simulink model "test_modelu"  (R2016a)
settings: Solver=VariableStepAuto  StartTime=0.0  StopTime=10.0  RelTol=1e-3
values from neighbouring files (symbols this model uses):
  A_dw = 110.74    [zmienne.m]
  A_fm = 59900/3    (= 19966.6666667)    [zmienne.m]
  A_fs = 60.67    [zmienne.m]
  A_p = (PI * (D_i^2) * N) / (4 * 144)    (= 11.0984259136)    [zmienne.m]
  alfa_c = -2.0 * 10^-4    (= -0.0002)    [zmienne.m]
  alfa_f = -1.1 * 10^-5    (= -1.1e-05)    [zmienne.m]
  B_1 = 0.000209    [zmienne.m]
  B_2 = 0.001414    [zmienne.m]
  B_3 = 0.001309    [zmienne.m]
  B_4 = 0.002727    [zmienne.m]
  B_5 = 0.000925    [zmienne.m]
  B_6 = 0.000314    [zmienne.m]
  B_t = 0.00689    [zmienne.m]
  C_1 = 1 / sqrt(C_d)    [zmienne.m]
  C_m = 0.11    [zmienne.m]
  C_p1 = 1.39    [zmienne.m]
  C_p2 = 1.165    [zmienne.m]
  C_pf = 0.059    [zmienne.m]
  C_pmo = 1.39    [zmienne.m]
  CP_fw = 1.218    [zmienne.m]
  DENS_d = 50.32    [zmienne.m]
  DENS_dw = 47.66    [zmienne.m]
  DENS_s = 52.32    [zmienne.m]
  DENS_w = 45.710    (= 45.71)    [zmienne.m]
  F_r = 0.974    [zmienne.m]
  G_1 = 65.2    [zmienne.m]
  G_2 = 1.0    (= 1)    [zmienne.m]
  G_v = 32.2    [zmienne.m]
  H_fm = 200/3600    (= 0.0555555555556)    [zmienne.m]
  K1 = 3.5 * 10^-6    (= 3.5e-06)    [zmienne.m]
  K2 = -7.135 * 10^-4    (= -0.0007135)    [zmienne.m]
  K3 = 0.17    [zmienne.m]
  K4 = -0.2    [zmienne.m]
  K5 = 0.14    [zmienne.m]
  K7 = 2.37 * 10^-3    (= 0.00237)    [zmienne.m]
  K9 = -0.035    [zmienne.m]
  L = 35.54    [zmienne.m]
  L_d = 35.54    [zmienne.m]
  L_dw0 = 9.63    [zmienne.m]
  L_r = 9.63    [zmienne.m]
  lambda_1 = 0.0125    [zmienne.m]
  lambda_2 = 0.0308    [zmienne.m]
  lambda_3 = 0.114    [zmienne.m]
  lambda_4 = 0.307    [zmienne.m]
  lambda_5 = 1.19    [zmienne.m]
  lambda_6 = 3.19    [zmienne.m]
  m0 = 0    [zmienne.m]
  M_d = DENS_d * A_d *L_d    (= 57227.9296)    [zmienne.m]
  M_f = M_ft * 3    (= 668217)    [zmienne.m]
  M_m1 = (M_m * L_s10) / L    (= 5577.64460636)    [zmienne.m]
  M_m2 = M_m * (L_s20 / L)    (= 51851.8797758)    [zmienne.m]
  M_m3 = M_m2    (= 51851.8797758)    [zmienne.m]
  M_m4 = M_m1    (= 5577.64460636)    [zmienne.m]
  M_mo = V_mo * DENS_mo / 3    (= 8227.8)    [zmienne.m]
  M_p1 = (M_p * L_s10) / L    (= 1751.07864275)    [zmienne.m]
  M_p2 = (M_p * L_s20) / L    (= 16278.6849414)    [zmienne.m]
  NGT = 17.9 * 10^-6    (= 1.79e-05)    [zmienne.m]
  P_0 = (P_cor10 * 3.41) / (3600 * 3)    (= 1084885.18519)    [zmienne.m]
  P_r2 = S_pm2 / L_s20    (= 687.386379167)    [zmienne.m]
  POWER_i = 691244.4199    [zmienne.m]
  r0 = 0    [zmienne.m]
  S_ms1 = S_m * (L_s10 / L)    (= 2678.800154)    [zmienne.m]
  S_ms2 = S_m * (L_s20 / L)    (= 24903.1326539)    [zmienne.m]
  S_ms3 = S_ms2    (= 24903.1326539)    [zmienne.m]
  S_ms4 = S_ms1    (= 2678.800154)    [zmienne.m]
  S_pm1 = (S_ms1 * D_i) / D_o    (= 2372.65156497)    [zmienne.m]
  S_pm2 = (S_ms2 * D_i) / D_o    (= 22057.0603506)    [zmienne.m]
  S_pm3 = S_pm1    (= 2372.65156497)    [zmienne.m]
  S_pm4 = S_pm2    (= 22057.0603506)    [zmienne.m]
  T_f10 = 1488.75    [zmienne.m]
  T_f20 = 1506.38    [zmienne.m]
  T_f30 = 1523.96    [zmienne.m]
  T_mo10 = 548.303    [zmienne.m]
  T_mo20 = 557.106    [zmienne.m]
  T_mo30 = 565.909    [zmienne.m]
  T_mo40 = 574.711    [zmienne.m]
  T_mo50 = 583.514    [zmienne.m]
  T_mo60 = 592.5    [zmienne.m]
  tau = 5    [zmienne.m]
  tau_1 = 250    [zmienne.m]
  tau_2 = 120    [zmienne.m]
  tau_cl = M_cl / W_pt    (= 2.08881752232)    [zmienne.m]
  tau_hl = M_hl / W_pt    (= 1.04440876116)    [zmienne.m]
  tau_la1 = 10    [zmienne.m]
  tau_la2 = 5    [zmienne.m]
  tau_le = 80    [zmienne.m]
  tau_lp = M_lp / W_pt    (= 1.87053609124)    [zmienne.m]
  tau_mo = M_mo / (2 * W_pt)    (= 0.0939967885046)    [zmienne.m]
  tau_pi = M_pi / W_pi    (= 0.60183806901)    [zmienne.m]
  tau_rtd = 4    [zmienne.m]
  tau_set = 30    [zmienne.m]
  tau_up = M_up / W_pt    (= 1.43710645536)    [zmienne.m]
  U_ms1 = 1 / (((1 / h_os) + (D_o * log(D_o/D_m))) / (24 * K_th))    [zmienne.m]
  U_ms2 = 1 / (((1 / h_ob) + (D_o * log(D_o/D_m))) / (24 * K_th))    [zmienne.m]
  U_pm = 1 / (((1 / h_i) + (D_i * log(D_m/D_i))) / (24 * K_th))    [zmienne.m]
  V_dr = 4398.706    [zmienne.m]
  V_r = 468.981    [zmienne.m]
  w0 = 0    [zmienne.m]
  W_fi0 = 1036.39    [zmienne.m]
  W_nv = 0.63    [zmienne.m]
  W_pi = 10941.6    [zmienne.m]
  X1 = 402.94    [zmienne.m]
  X2 = 0.018    [zmienne.m]
  X3 = 1.13096    [zmienne.m]
  X4 = 370.751    [zmienne.m]
  X5 = 850.04    [zmienne.m]
  X6 = -0.181289    [zmienne.m]
  X8 = 1225.85    [zmienne.m]
  Z_tv = 3.18    [zmienne.m]
undefined symbols (not defined in the file or in its folder): magnitude
(part 1 of 2)
settings Model: Creator=Użytkownik  LastModifiedBy=Użytkownik
settings GRTTargetCC: GeneratePreprocessorConditionals=Use local settings

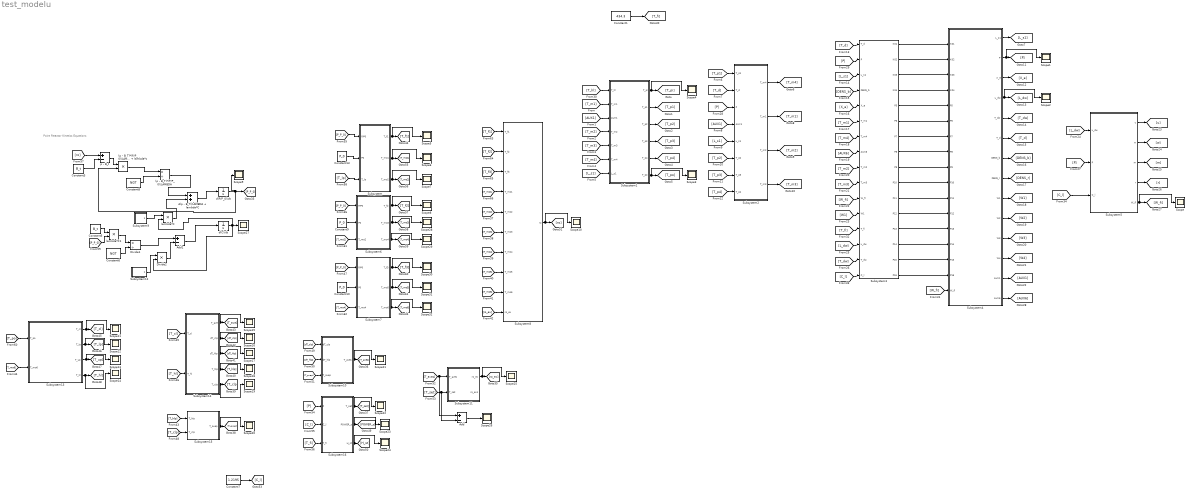
== system test_modelu ==
  note: Point Reactor Kinetics Equations
  (p - B_T)*(P/P_0)/LAMBDA : Product  Inputs=*/
  (p - B_T)*(P/P_0)/LAMBDA + lambda*c : Product  Inputs=**
  A(p - B_T)/LAMBDA + lambda*C : Sum
  Add : Sum  Inputs=+-
  Add1 : Sum  Inputs=+-
  Constant1 : Constant  Value=434.3
  Constant10 : Constant  Value=P_0
  Constant13 : Constant  Value=P_0
  Constant3 : Constant  Value=B_t
  Constant5 : Constant  Value=B_t
  Constant6 : Constant  Value=NGT
  Constant7 : Constant  Value=1.2195
  Constant8 : Constant  Value=NGT
  Constant9 : Constant  Value=P_0
  Divide1 : Product  Inputs=*/
  Divide2 : Product  Inputs=**
  Scope{,1..32} (33 alike) : Scope
  Subsystem : Subsystem
  Subsystem1 : Subsystem
  Subsystem10 : Subsystem
  Subsystem11 : Subsystem
  Subsystem12 : Subsystem
  Subsystem13 : Subsystem
  Subsystem14 : Subsystem
  Subsystem15 : Subsystem
  Subsystem16 : Subsystem
  Subsystem2 : Subsystem
  Subsystem3 : Subsystem
  Subsystem4 : Subsystem
  Subsystem5 : Subsystem
  Subsystem6 : Subsystem
  Subsystem7 : Subsystem
  Subsystem8 : Subsystem
  Subsystem9 : Subsystem
  d(C)/dt : Integrator  InitialCondition=4625.71
  d(P/P_0)/dt : Integrator  InitialCondition=1
  lambda*C : Product  Inputs=**
  lambda*C1 : Product  Inputs=**
  p - B_t : Sum  Inputs=+-
  wires:
  Subsystem1/1(T_pi) -> Scope4/1, [T_pi]
  Subsystem1/2(T_p1) -> [T_p1]
  Subsystem1/3(T_p2) -> [T_p2]
  Subsystem1/4(T_p3) -> [T_p3]
  Subsystem1/5(T_p4) -> [T_p4]
  Subsystem1/6(T_po) -> Scope3/1, [T_po]
  Subsystem2/1(T_m4) -> [T_m4]
  Subsystem2/2(T_m1) -> [T_m1]
  Subsystem2/3(T_m2) -> [T_m2]
  Subsystem2/4(T_m3) -> [T_m3]
  Subsystem4/1(L_s1) -> [L_s1]
  Subsystem4/2(P) -> Scope1/1, [P]
  Subsystem4/3(X_e) -> [X_e]
  Subsystem4/4(L_dw) -> Scope2/1, [L_dw]
  Subsystem4/5(T_dw) -> [T_dw]
  Subsystem4/6(T_d) -> [T_d]
  Subsystem4/7(DENS_b) -> [DENS_b]
  Subsystem4/8(DENS_r) -> [DENS_r]
  Subsystem4/9(W1) -> [W1]
  Subsystem4/10(W2) -> [W2]
  Subsystem4/11(W3) -> [W3]
  Subsystem4/12(W4) -> [W4]
  Subsystem4/13(AUX1) -> [AUX1]
  [T_m1] -> Subsystem1/2(T_m1)
  [AUX1] -> Subsystem1/3(AUX1)
  [T_m2] -> Subsystem1/4(T_m2)
  [T_m3] -> Subsystem1/5(T_m3)
  [T_m4] -> Subsystem1/6(T_m4)
  [L_s1] -> Subsystem1/7(L_s1)
  Subsystem5/1(u) -> [u]
  Subsystem5/2(w) -> [w]
  Subsystem5/3(m) -> [m]
  Subsystem5/4(r) -> [r]
  Subsystem5/5(W_fi) -> Scope/1, [W_fi]
  [T_p1] -> Subsystem2/1(T_p1)
  [T_d] -> Subsystem2/2(T_d)
  [AUX1] -> Subsystem2/4(AUX1)
  [L_s1] -> Subsystem2/5(L_s1)
  [T_p2] -> Subsystem2/6(T_p2)
  [T_p3] -> Subsystem2/7(T_p3)
  [T_p4] -> Subsystem2/8(T_p4)
  [T_d] -> Subsystem3/1(T_d)
  [L_s1] -> Subsystem3/3(L_s1)
  [DENS_b] -> Subsystem3/4(DENS_b)
  [X_e] -> Subsystem3/5(X_e)
  [T_m1] -> Subsystem3/6(T_m1)
  [T_m4] -> Subsystem3/7(T_m4)
  [T_m2] -> Subsystem3/9(T_m2)
  [T_m3] -> Subsystem3/10(T_m3)
  [W_fi] -> Subsystem3/11(W_fi)
  [AUX6] -> Subsystem3/8(AUX6)
  Subsystem4/14(AUX6) -> [AUX6]
  [W1] -> Subsystem3/12(W1)
  [L_dw] -> Subsystem3/14(L_dw)
  [T_dw] -> Subsystem3/15(T_dw)
  [L_dw] -> Subsystem5/1(L_dw)
  [P] -> Subsystem5/2(P)
  [P] -> Subsystem2/3(P)
  [P] -> Subsystem3/2(P)
  [T_hl] -> Subsystem1/1(T_hl)
  [W_fi] -> Subsystem4/17(W_fi)
  [T_fi] -> Subsystem3/13(T_fi)
  [C_l] -> Subsystem3/16(C_l)
  [C_l] -> Subsystem5/3(C_l)
  Constant1/1 -> [T_fi]
  Subsystem3/1(K01) -> Subsystem4/1(K01)
  Subsystem3/2(K02) -> Subsystem4/2(K02)
  Subsystem3/3(K03) -> Subsystem4/3(K03)
  Subsystem3/4("K04 ") -> Subsystem4/4(K04)
  Subsystem3/5(P5) -> Subsystem4/5(P5)
  Subsystem3/6(P6) -> Subsystem4/6(P6)
  Subsystem3/7(P7) -> Subsystem4/7(P7)
  Subsystem3/8(P8) -> Subsystem4/8(P8)
  Subsystem3/9(P9) -> Subsystem4/9(P9)
  Subsystem3/10(P10) -> Subsystem4/10(P10)
  Subsystem3/11(P11) -> Subsystem4/11(P11)
  Subsystem3/12(P12) -> Subsystem4/12(P12)
  Subsystem3/13(P13) -> Subsystem4/13(P13)
  Subsystem3/14(P14) -> Subsystem4/14(P14)
  Subsystem3/15(P15) -> Subsystem4/15(P15)
  Subsystem3/16(P16) -> Subsystem4/16(P16)
  Constant3/1 -> p - B_t/2
  Constant8/1 -> (p - B_T)*(P/P_0)/LAMBDA/2
  Subsystem9/1(lambda) -> lambda*C/1
  d(C)/dt/1 -> Scope27/1, Divide2/2, lambda*C/2
  lambda*C/1 -> A(p - B_T)/LAMBDA + lambda*C/2
  A(p - B_T)/LAMBDA + lambda*C/1 -> d(P/P_0)/dt/1
  Constant6/1 -> Divide1/2
  Divide1/1 -> Add1/1
  Subsystem12/1(lambda) -> Divide2/1
  Divide2/1 -> Add1/2
  Add1/1 -> d(C)/dt/1
  d(P/P_0)/dt/1 -> (p - B_T)*(P/P_0)/LAMBDA + lambda*c/2, [P_P_0], Scope9/1
  Constant13/1 -> Subsystem/2(P0)
  Constant9/1 -> Subsystem6/2(P0)
  Constant10/1 -> Subsystem7/2(P0)
  [T_po] -> Subsystem13/1(T_po)
  [P_P_0] -> Subsystem/1("P/P0 ")
  [P_P_0] -> Subsystem6/1("P/P0 ")
  [P_P_0] -> Subsystem7/1("P/P0 ")
  Subsystem/1(T_f1) -> Scope5/1, [T_f1]
  Subsystem/2(T_mo1) -> Scope6/1, [T_mo1]
  Subsystem/3(T_mo2) -> Scope7/1, [T_mo2]
  Subsystem6/1(T_f2) -> Scope8/1, [T_f2]
  Subsystem6/2(T_mo3) -> Scope28/1, [T_mo3]
  Subsystem6/3(T_mo4) -> Scope29/1, [T_mo4]
  Subsystem7/1(T_f3) -> Scope30/1, [T_f3]
  Subsystem7/2(T_mo5) -> Scope31/1, [T_mo5]
  Subsystem7/3(T_mo6) -> Scope32/1, [T_mo6]
  [T_lp] -> Subsystem/3(T_lp)
  [T_mo2] -> Subsystem6/3(T_mo2)
  [T_mo4] -> Subsystem7/3(T_mo4)
  [T_f1] -> Subsystem8/1(T_f1)
  [T_f2] -> Subsystem8/2(T_f2)
  [T_f3] -> Subsystem8/3(T_f3)
  [T_mo1] -> Subsystem8/4(T_mo1)
  [T_mo2] -> Subsystem8/5(T_mo2)
  [T_mo3] -> Subsystem8/6(T_mo3)
  [T_mo4] -> Subsystem8/7(T_mo4)
  [T_mo5] -> Subsystem8/8(T_mo5)
  [T_mo6] -> Subsystem8/9(T_mo6)
  [ro_ex] -> Subsystem8/10(ro_ex)
  [T_cl] -> Subsystem14/1(T_cl)
  [T_hl] -> Subsystem14/2(T_hl)
  [T_hlp] -> Subsystem15/1(T_hlp)
  [T_clp] -> Subsystem15/2(T_clp)
  [dT_clp] -> Subsystem10/1(dT_clp)
  [dT_hlp] -> Subsystem10/2(dT_hlp)
  [T_avep] -> Subsystem10/3(T_avep)
  [T_aves] -> Add/1, Subsystem11/1(T_aves)
  [T_set] -> Add/2, Subsystem11/2(T_set)
  Subsystem10/1(T_aves) -> Scope21/1, [T_aves]
  Subsystem16/1(T_set) -> Scope22/1, [T_set]
  Subsystem15/1(T_avep) -> Scope20/1, [T_avep]
  Subsystem14/5(T_clp) -> Scope19/1, [T_clp]
  Subsystem14/4(T_hlp) -> Scope18/1, [T_hlp]
  Subsystem14/3(dT_hlp) -> Scope17/1, [dT_hlp]
  Subsystem14/2(dT_clp) -> Scope16/1, [dT_clp]
  Subsystem14/1(T_ave) -> Scope15/1, [T_ave]
  Subsystem13/3(T_up) -> Scope13/1, [T_up]
  Subsystem13/2(T_lp) -> Scope12/1, [T_lp]
  Subsystem13/1(T_cl) -> Scope11/1, [T_cl]
  Subsystem16/2(POWER_s) -> [POWER_s], Scope23/1
  [P] -> Subsystem16/1(P)
  [C_l] -> Subsystem16/2(C_l)
  [T_fi] -> Subsystem16/3(T_fi)
  [T_mo6] -> Subsystem13/2(T_mo6)
  Subsystem8/1(ro) -> Scope10/1, [ro]
  Constant7/1 -> [C_l]
  Constant5/1 -> lambda*C1/1
  [P_P_0] -> lambda*C1/2
  lambda*C1/1 -> Divide1/1
  Subsystem11/1(ro_ex) -> Scope25/1, [ro_ex]
  Subsystem16/3(H_st) -> Scope24/1, [H_st]
  Add/1 -> Scope26/1
  Subsystem13/4(T_hl) -> Scope14/1, [T_hl]
  p - B_t/1 -> (p - B_T)*(P/P_0)/LAMBDA + lambda*c/1
  (p - B_T)*(P/P_0)/LAMBDA + lambda*c/1 -> (p - B_T)*(P/P_0)/LAMBDA/1
  (p - B_T)*(P/P_0)/LAMBDA/1 -> A(p - B_T)/LAMBDA + lambda*C/1
  [ro] -> p - B_t/1

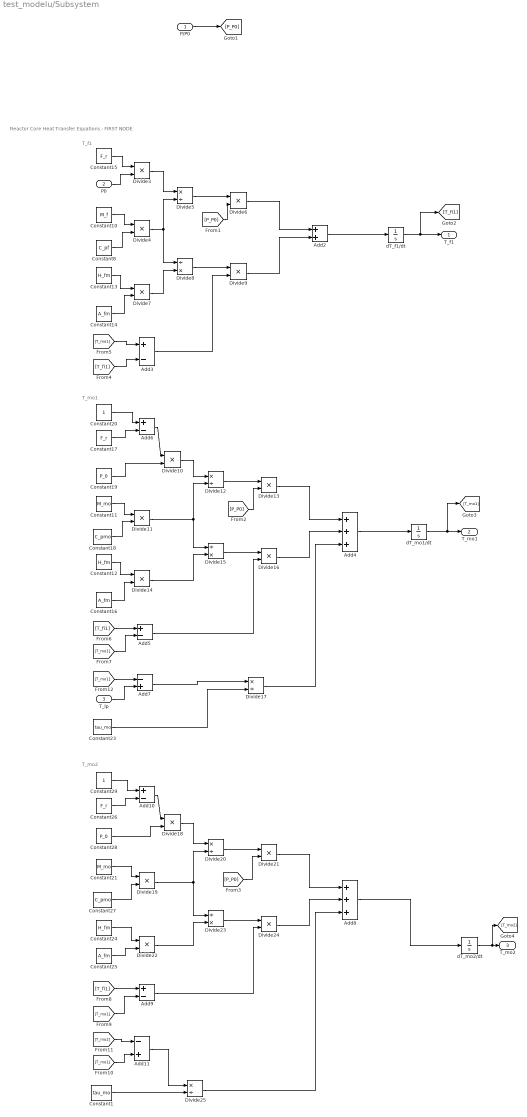
== system test_modelu/Subsystem ==
  note: T_mo2
  note: T_mo1
  note: T_f1
  note: Reactor Core Heat Transfer Equations : FIRST NODE
  "P/P0 " : Inport
  P0 : Inport  Port=2
  T_lp : Inport  Port=3
  Add{3,5..6,9..10} (5 alike) : Sum  Inputs=+-
  Add11 : Sum  Inputs=-+
  Add2 : Sum
  Add4 : Sum  Inputs=+++
  Add7 : Sum  Inputs=-+
  Add8 : Sum  Inputs=+++
  Constant1 : Constant  Value=tau_mo
  Constant10 : Constant  Value=M_f
  Constant11 : Constant  Value=M_mo
  Constant12 : Constant  Value=H_fm
  Constant13 : Constant  Value=H_fm
  Constant14 : Constant  Value=A_fm
  Constant15 : Constant  Value=F_r
  Constant16 : Constant  Value=A_fm
  Constant17 : Constant  Value=F_r
  Constant18 : Constant  Value=C_pmo
  Constant19 : Constant  Value=P_0
  Constant20 : Constant
  Constant21 : Constant  Value=M_mo
  Constant23 : Constant  Value=tau_mo
  Constant24 : Constant  Value=H_fm
  Constant25 : Constant  Value=A_fm
  Constant26 : Constant  Value=F_r
  Constant27 : Constant  Value=C_pmo
  Constant28 : Constant  Value=P_0
  Constant29 : Constant
  Constant8 : Constant  Value=C_pf
  Divide{3..4,6..7,9..11,13..14,16,18..19,21..22,24} (15 alike) : Product  Inputs=**
  Divide{5,12,17,20,25} (5 alike) : Product  Inputs=*/
  Divide15 : Product  Inputs=/*
  Divide23 : Product  Inputs=/*
  Divide8 : Product  Inputs=/*
  dT_f1/dt : Integrator  InitialCondition=1488.75
  dT_mo1/dt : Integrator  InitialCondition=548.303
  dT_mo2/dt : Integrator  InitialCondition=557.106
  T_f1 : Outport
  T_mo1 : Outport  Port=2
  T_mo2 : Outport  Port=3
  wires:
  Constant15/1 -> Divide3/1
  Constant10/1 -> Divide4/1
  Constant8/1 -> Divide4/2
  Divide3/1 -> Divide5/1
  Divide4/1 -> Divide5/2, Divide8/1
  Divide5/1 -> Divide6/1
  Divide6/1 -> Add2/1
  Constant13/1 -> Divide7/1
  Constant14/1 -> Divide7/2
  Divide7/1 -> Divide8/2
  Divide8/1 -> Divide9/1
  dT_mo1/dt/1 -> [T_mo1], T_mo1/1
  dT_f1/dt/1 -> [T_fi1], T_f1/1
  Add3/1 -> Divide9/2
  Divide9/1 -> Add2/2
  Add2/1 -> dT_f1/dt/1
  Constant19/1 -> Divide10/2
  Constant11/1 -> Divide11/1
  Constant18/1 -> Divide11/2
  Divide10/1 -> Divide12/1
  Divide11/1 -> Divide15/1, Divide12/2
  Divide12/1 -> Divide13/1
  Divide13/1 -> Add4/1
  Constant12/1 -> Divide14/1
  Constant16/1 -> Divide14/2
  Divide14/1 -> Divide15/2
  Divide15/1 -> Divide16/1
  Add5/1 -> Divide16/2
  Divide16/1 -> Add4/2
  Constant20/1 -> Add6/1
  Constant17/1 -> Add6/2
  Add6/1 -> Divide10/1
  T_lp/1 -> Add7/2
  Add7/1 -> Divide17/1
  Constant23/1 -> Divide17/2
  Divide17/1 -> Add4/3
  Add4/1 -> dT_mo1/dt/1
  dT_mo2/dt/1 -> [T_mo2], T_mo2/1
  Constant28/1 -> Divide18/2
  Constant21/1 -> Divide19/1
  Constant27/1 -> Divide19/2
  Divide18/1 -> Divide20/1
  Divide19/1 -> Divide20/2, Divide23/1
  Divide20/1 -> Divide21/1
  Divide21/1 -> Add8/1
  Constant24/1 -> Divide22/1
  Constant25/1 -> Divide22/2
  Divide22/1 -> Divide23/2
  Divide23/1 -> Divide24/1
  Add9/1 -> Divide24/2
  Divide24/1 -> Add8/2
  Constant29/1 -> Add10/1
  Constant26/1 -> Add10/2
  Add10/1 -> Divide18/1
  Add11/1 -> Divide25/1
  Divide25/1 -> Add8/3
  Add8/1 -> dT_mo2/dt/1
  "P/P0 "/1 -> [P_P0]
  P0/1 -> Divide3/2
  [P_P0] -> Divide6/2
  [P_P0] -> Divide21/2
  [P_P0] -> Divide13/2
  [T_mo1] -> Add3/1
  [T_fi1] -> Add3/2
  [T_fi1] -> Add5/1
  [T_mo1] -> Add5/2
  [T_fi1] -> Add9/1
  [T_mo1] -> Add9/2
  [T_mo2] -> Add11/1
  [T_mo1] -> Add11/2
  [T_mo1] -> Add7/1
  Constant1/1 -> Divide25/2

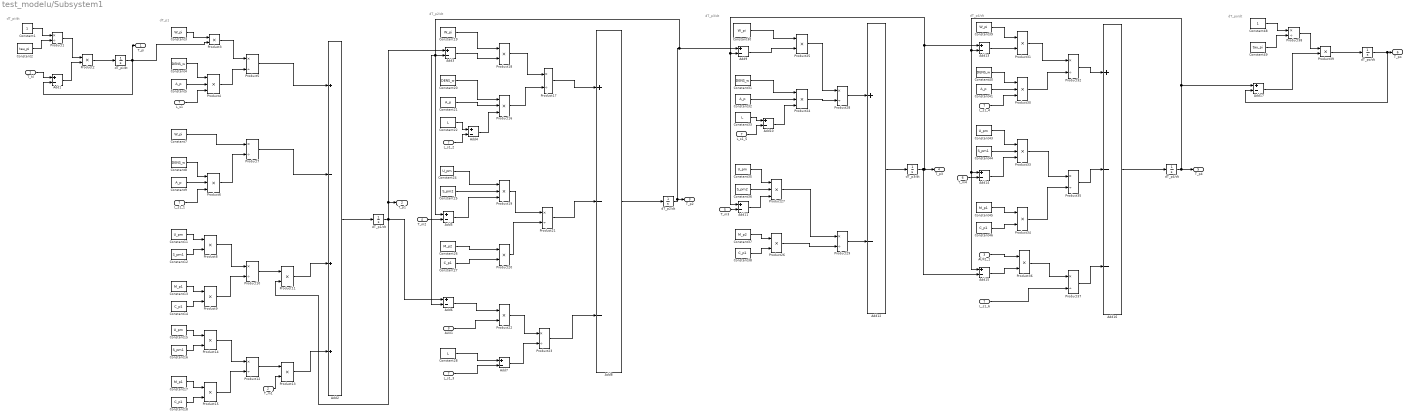
== system test_modelu/Subsystem1 ==
  note: dT_po/dt
  note: dT_p4/dt
  note: dT_p3/dt
  note: dT_p2/dt
  note: dT_p1
  note: dT_pi/dt
  T_hl : Inport
  T_m1 : Inport  Port=2
  AUX1 : Inport  Port=3
  T_m2 : Inport  Port=4
  T_m3 : Inport  Port=5
  T_m4 : Inport  Port=6
  L_s1 : Inport  Port=7
  AUX1_1 : InportShadow  Port=3
  Add{1,3..7,9..15,17} (14 alike) : Sum  Inputs=+-
  Add16 : Sum  Inputs=+--
  Add2 : Sum  Inputs=+-++
  Add8 : Sum  Inputs=+--
  Constant1 : Constant
  Constant{11,15,24,35,43} (5 alike) : Constant  Value=U_pm
  Constant12 : Constant  Value=S_pm1
  Constant13 : Constant  Value=M_p1
  Constant{14,18,27,38,46} (5 alike) : Constant  Value=C_p1
  Constant16 : Constant  Value=S_pm1
  Constant17 : Constant  Value=M_p1
  Constant{3,7,19,30,39} (5 alike) : Constant  Value=W_pi
  Constant2 : Constant  Value=tau_pi
  Constant{4,8,20,31,40} (5 alike) : Constant  Value=DENS_w
  Constant{5,9,21,32,41} (5 alike) : Constant  Value=A_p
  Constant22 : Constant  Value=L
  Constant25 : Constant  Value=S_pm2
  Constant26 : Constant  Value=M_p2
  Constant28 : Constant  Value=L
  Constant33 : Constant  Value=L
  Constant36 : Constant  Value=S_pm2
  Constant37 : Constant  Value=M_p2
  Constant44 : Constant  Value=S_pm1
  Constant45 : Constant  Value=M_p1
  Constant48 : Constant
  Constant49 : Constant  Value=tau_pi
  L_s1_{1..6} (6 alike) : InportShadow  Port=7
  Product{1,5,7,10,12,17,21,23,28..29,32,35,37..38} (14 alike) : Product  Inputs=*/
  Product{2..3,8..9,11,13..15,18,20,22,25..26,31,34,36,39} (17 alike) : Product
  Product{4,6,16,19,24,27,30,33} (8 alike) : Product  Inputs=3
  dT_p1/dt : Integrator  InitialCondition=587.36
  dT_p2/dt : Integrator  InitialCondition=557.4
  dT_p3/dt : Integrator  InitialCondition=542.5
  dT_p4/dt : Integrator  InitialCondition=539.5
  dT_pi/dt : Integrator  InitialCondition=592.5
  dT_po/dt : Integrator  InitialCondition=539.5
  T_pi : Outport
  T_p1 : Outport  Port=2
  T_p2 : Outport  Port=3
  T_p3 : Outport  Port=4
  T_p4 : Outport  Port=5
  T_po : Outport  Port=6
  wires:
  Constant1/1 -> Product1/1
  Constant2/1 -> Product1/2
  T_hl/1 -> Add1/1
  Product1/1 -> Product2/1
  Add1/1 -> Product2/2
  Product2/1 -> dT_pi/dt/1
  dT_pi/dt/1 -> T_pi/1, Product3/2, Add1/2
  Constant3/1 -> Product3/1
  Constant4/1 -> Product4/1
  Constant5/1 -> Product4/2
  L_s1/1 -> Product4/3
  Product3/1 -> Product5/1
  Product4/1 -> Product5/2
  Constant8/1 -> Product6/1
  Constant9/1 -> Product6/2
  L_s1_1/1 -> Product6/3
  Constant7/1 -> Product7/1
  Product6/1 -> Product7/2
  Constant11/1 -> Product8/1
  Constant12/1 -> Product8/2
  Constant13/1 -> Product9/1
  Constant14/1 -> Product9/2
  Product8/1 -> Product10/1
  Product9/1 -> Product10/2
  Product10/1 -> Product11/1
  Constant15/1 -> Product14/1
  Constant16/1 -> Product14/2
  Constant17/1 -> Product15/1
  Constant18/1 -> Product15/2
  Product14/1 -> Product12/1
  Product15/1 -> Product12/2
  Product12/1 -> Product13/1
  T_m1/1 -> Product13/2
  Product5/1 -> Add2/1
  Product7/1 -> Add2/2
  Product11/1 -> Add2/3
  Product13/1 -> Add2/4
  dT_p1/dt/1 -> Add6/1, Product11/2, T_p1/1, Add3/1
  Add2/1 -> dT_p1/dt/1
  Constant22/1 -> Add4/1
  L_s1_2/1 -> Add4/2
  Constant20/1 -> Product16/1
  Constant21/1 -> Product16/2
  Add4/1 -> Product16/3
  Constant19/1 -> Product18/1
  Add3/1 -> Product18/2
  Product18/1 -> Product17/1
  Product16/1 -> Product17/2
  Add5/1 -> Product19/3
  Constant25/1 -> Product19/2
  Constant24/1 -> Product19/1
  Constant26/1 -> Product20/1
  Constant27/1 -> Product20/2
  Product19/1 -> Product21/1
  Product20/1 -> Product21/2
  dT_p2/dt/1 -> T_p2/1, Add5/1, Add3/2, Add6/2, Add9/1
  Add6/1 -> Product22/1
  AUX1/1 -> Product22/2
  Constant28/1 -> Add7/1
  L_s1_3/1 -> Add7/2
  Product22/1 -> Product23/1
  Add7/1 -> Product23/2
  Add8/1 -> dT_p2/dt/1
  Product17/1 -> Add8/1
  Product21/1 -> Add8/2
  Product23/1 -> Add8/3
  Constant33/1 -> Add10/1
  L_s1_5/1 -> Add10/2
  Constant31/1 -> Product24/1
  Constant32/1 -> Product24/2
  Add10/1 -> Product24/3
  Constant30/1 -> Product25/1
  Add9/1 -> Product25/2
  dT_p3/dt/1 -> T_p3/1, Add11/1, Add9/2, Add13/1, Add15/2
  Constant37/1 -> Product26/1
  Constant38/1 -> Product26/2
  Constant35/1 -> Product27/1
  Constant36/1 -> Product27/2
  Add11/1 -> Product27/3
  T_m2/1 -> Add5/2
  T_m3/1 -> Add11/2
  Add12/1 -> dT_p3/dt/1
  Product28/1 -> Add12/1
  Product25/1 -> Product28/1
  Product24/1 -> Product28/2
  Product29/1 -> Add12/2
  Product27/1 -> Product29/1
  Product26/1 -> Product29/2
  dT_p4/dt/1 -> T_p4/1, Add17/1, Add15/1, Add14/1, Add13/2
  Constant41/1 -> Product30/2
  Constant40/1 -> Product30/1
  L_s1_4/1 -> Product30/3
  Constant39/1 -> Product31/1
  Add13/1 -> Product31/2
  Product31/1 -> Product32/1
  Product30/1 -> Product32/2
  T_m4/1 -> Add14/2
  Constant43/1 -> Product33/1
  Constant44/1 -> Product33/2
  Add14/1 -> Product33/3
  Constant45/1 -> Product34/1
  Constant46/1 -> Product34/2
  Product33/1 -> Product35/1
  Product34/1 -> Product35/2
  AUX1_1/1 -> Product36/1
  Add15/1 -> Product36/2
  Product36/1 -> Product37/1
  L_s1_6/1 -> Product37/2
  Add16/1 -> dT_p4/dt/1
  Product32/1 -> Add16/1
  Product35/1 -> Add16/2
  Product37/1 -> Add16/3
  Constant48/1 -> Product38/1
  Constant49/1 -> Product38/2
  dT_po/dt/1 -> Add17/2, T_po/1
  Product38/1 -> Product39/1
  Add17/1 -> Product39/2
  Product39/1 -> dT_po/dt/1

== system test_modelu/Subsystem10 ==
  dT_clp : Inport
  dT_hlp : Inport  Port=2
  T_avep : Inport  Port=3
  Add : Sum  Inputs=+--+
  Add1 : Sum
  Add2 : Sum
  Constant1 : Constant  Value=tau_la1
  Constant2 : Constant  Value=tau_la2
  Constant3 : Constant  Value=tau_le
  Constant4 : Constant  Value=2
  Constant5 : Constant  Value=tau_la1
  Constant6 : Constant  Value=tau_la2
  Divide : Product  Inputs=*/
  Divide1 : Product  Inputs=**
  Divide2 : Product  Inputs=*/
  Divide3 : Product  Inputs=**
  Divide4 : Product  Inputs=**
  dT_aves/dt : Integrator  InitialCondition=566
  d^2T_aves/dt : Integrator
  T_aves : Outport
  wires:
  T_avep/1 -> Add/1
  dT_aves/dt/1 -> [T_aves], T_aves/1
  Constant1/1 -> Add1/1
  Constant2/1 -> Add1/2
  Add1/1 -> Divide1/1
  d^2T_aves/dt/1 -> [AUX_co], dT_aves/dt/1
  Divide1/1 -> Add/3
  dT_clp/1 -> Add2/1
  dT_hlp/1 -> Add2/2
  Add2/1 -> Divide2/1
  Constant4/1 -> Divide2/2
  Constant3/1 -> Divide3/1
  Divide2/1 -> Divide3/2
  Divide3/1 -> Add/4
  Constant5/1 -> Divide4/1
  Constant6/1 -> Divide4/2
  Divide4/1 -> Divide/2
  Add/1 -> Divide/1
  Divide/1 -> d^2T_aves/dt/1
  [AUX_co] -> Divide1/2
  [T_aves] -> Add/2

== system test_modelu/Subsystem11 ==
  T_aves : Inport
  T_set : Inport  Port=2
  Integrator : Integrator
  MATLAB Function : MATLAB Function  TreatAsAtomicUnit=on
  MATLAB Function1 : MATLAB Function  TreatAsAtomicUnit=on
  Scope : Scope  NumInputPorts=2
  Scope1 : Scope
  Scope2 : Scope
  Scope3 : Scope
  ro_ex : Outport
  ro_ex1 : Outport  Port=2
  wires:
  T_set/1 -> MATLAB Function/1(u1)
  T_aves/1 -> MATLAB Function/2(u2)
  MATLAB Function/1(y1) -> Scope/2, Scope2/1, Integrator/1
  Integrator/1 -> Scope3/1, MATLAB Function1/1(u), ro_ex/1, Scope/1
  MATLAB Function1/1(y) -> Scope1/1, ro_ex1/1

== system test_modelu/Subsystem12 ==
  Add : Sum  Inputs=++++++
  Constant : Constant  Value=B_t
  Constant1 : Constant  Value=B_1
  Constant10 : Constant  Value=lambda_5
  Constant11 : Constant  Value=lambda_6
  Constant12 : Constant  Value=B_6
  Constant2 : Constant  Value=lambda_1
  Constant3 : Constant  Value=B_2
  Constant4 : Constant  Value=lambda_2
  Constant5 : Constant  Value=B_3
  Constant6 : Constant  Value=lambda_3
  Constant7 : Constant  Value=B_4
  Constant8 : Constant  Value=lambda_4
  Constant9 : Constant  Value=B_5
  Divide{,1..6} (7 alike) : Product  Inputs=*/
  lambda : Outport
  wires:
  Divide6/1 -> lambda/1
  Constant/1 -> Divide6/1
  Add/1 -> Divide6/2
  Divide/1 -> Add/1
  Divide2/1 -> Add/3
  Divide1/1 -> Add/2
  Divide3/1 -> Add/4
  Divide4/1 -> Add/5
  Divide5/1 -> Add/6
  Constant11/1 -> Divide5/2
  Constant12/1 -> Divide5/1
  Constant10/1 -> Divide4/2
  Constant9/1 -> Divide4/1
  Constant8/1 -> Divide3/2
  Constant7/1 -> Divide3/1
  Constant6/1 -> Divide2/2
  Constant5/1 -> Divide2/1
  Constant4/1 -> Divide1/2
  Constant3/1 -> Divide1/1
  Constant2/1 -> Divide/2
  Constant1/1 -> Divide/1

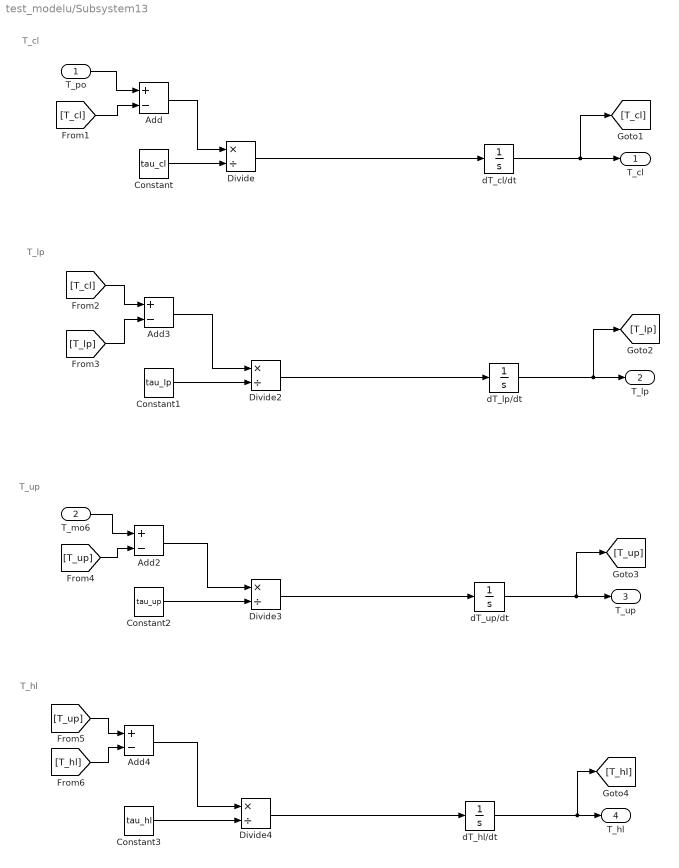
== system test_modelu/Subsystem13 ==
  note: T_hl
  note: T_up
  note: T_lp
  note: T_cl
  T_po : Inport
  T_mo6 : Inport  Port=2
  Add{,2..4} (4 alike) : Sum  Inputs=+-
  Constant : Constant  Value=tau_cl
  Constant1 : Constant  Value=tau_lp
  Constant2 : Constant  Value=tau_up
  Constant3 : Constant  Value=tau_hl
  Divide{,2..4} (4 alike) : Product  Inputs=*/
  dT_cl/dt : Integrator  InitialCondition=539.5
  dT_hl/dt : Integrator  InitialCondition=592.5
  dT_lp/dt : Integrator  InitialCondition=539.5
  dT_up/dt : Integrator  InitialCondition=592.5
  T_cl : Outport
  T_lp : Outport  Port=2
  T_up : Outport  Port=3
  T_hl : Outport  Port=4
  wires:
  T_po/1 -> Add/1
  dT_cl/dt/1 -> [T_cl], T_cl/1
  Constant/1 -> Divide/2
  Add/1 -> Divide/1
  Divide/1 -> dT_cl/dt/1
  Constant2/1 -> Divide3/2
  Divide2/1 -> dT_lp/dt/1
  Divide3/1 -> dT_up/dt/1
  Divide4/1 -> dT_hl/dt/1
  dT_lp/dt/1 -> [T_lp], T_lp/1
  T_mo6/1 -> Add2/1
  Add2/1 -> Divide3/1
  dT_up/dt/1 -> [T_up], T_up/1
  dT_hl/dt/1 -> [T_hl], T_hl/1
  Add4/1 -> Divide4/1
  Constant1/1 -> Divide2/2
  Constant3/1 -> Divide4/2
  Add3/1 -> Divide2/1
  [T_cl] -> Add/2
  [T_cl] -> Add3/1
  [T_lp] -> Add3/2
  [T_up] -> Add2/2
  [T_up] -> Add4/1
  [T_hl] -> Add4/2

== system test_modelu/Subsystem14 ==
  T_cl : Inport
  T_hl : Inport  Port=2
  Add : Sum
  Add1 : Sum  Inputs=+-
  Add2 : Sum  Inputs=+-
  Constant : Constant  Value=2
  Constant1 : Constant  Value=tau_rtd
  Constant2 : Constant  Value=tau_rtd
  dT_clp/dt1 : Integrator  InitialCondition=539.5
  dT_hlp/dt : Integrator  InitialCondition=592.5
  ss : Product  Inputs=*/
  ss1 : Product  Inputs=*/
  ss2 : Product  Inputs=*/
  T_ave : Outport
  dT_clp : Outport  Port=2
  dT_hlp : Outport  Port=3
  T_hlp : Outport  Port=4
  T_clp : Outport  Port=5
  wires:
  T_hl/1 -> Add1/1, Add/2
  Add/1 -> ss/1
  Constant/1 -> ss/2
  ss/1 -> T_ave/1
  dT_hlp/dt/1 -> Add1/2, T_hlp/1
  Add1/1 -> ss1/1
  Constant1/1 -> ss1/2
  ss1/1 -> dT_hlp/1, dT_hlp/dt/1
  T_cl/1 -> Add2/1, Add/1
  dT_clp/dt1/1 -> Add2/2, T_clp/1
  Add2/1 -> ss2/1
  Constant2/1 -> ss2/2
  ss2/1 -> dT_clp/1, dT_clp/dt1/1

== system test_modelu/Subsystem15 ==
  T_hlp : Inport
  T_clp : Inport  Port=2
  Add1 : Sum
  Constant4 : Constant  Value=2
  Divide1 : Product  Inputs=*/
  T_avep : Outport
  wires:
  T_hlp/1 -> Add1/1
  T_clp/1 -> Add1/2
  Add1/1 -> Divide1/1
  Constant4/1 -> Divide1/2
  Divide1/1 -> T_avep/1

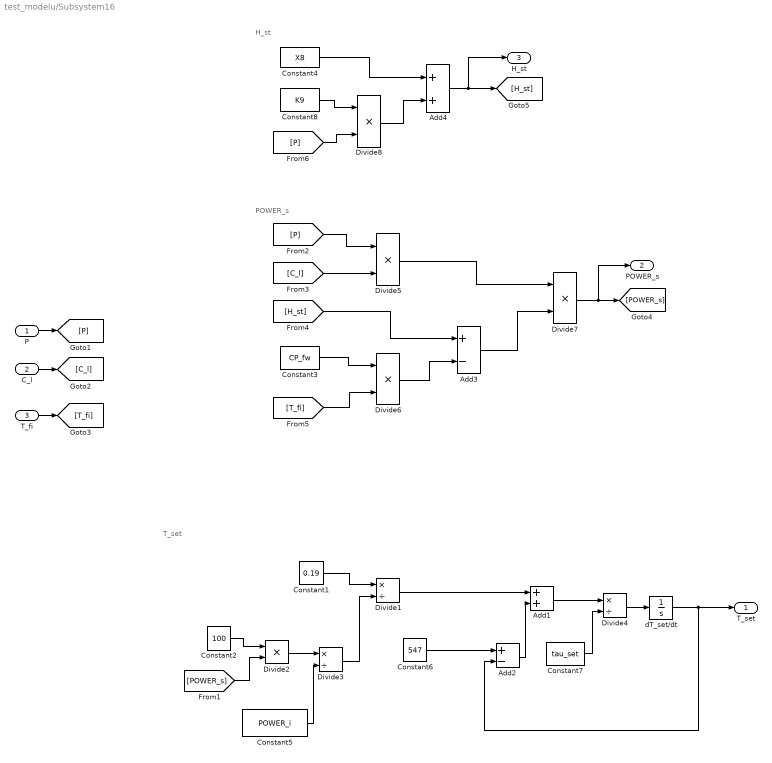
== system test_modelu/Subsystem16 ==
  note: H_st
  note: POWER_s
  note: T_set
  P : Inport
  C_l : Inport  Port=2
  T_fi : Inport  Port=3
  Add1 : Sum
  Add2 : Sum  Inputs=+-
  Add3 : Sum  Inputs=+-
  Add4 : Sum  Inputs=2
  Constant1 : Constant  Value=0.19
  Constant2 : Constant  Value=100
  Constant3 : Constant  Value=CP_fw
  Constant4 : Constant  Value=X8
  Constant5 : Constant  Value=POWER_i
  Constant6 : Constant  Value=547
  Constant7 : Constant  Value=tau_set
  Constant8 : Constant  Value=K9
  Divide1 : Product  Inputs=*/
  Divide2 : Product  Inputs=**
  Divide3 : Product  Inputs=*/
  Divide4 : Product  Inputs=*/
  Divide{5..8} (4 alike) : Product
  dT_set/dt : Integrator  InitialCondition=566
  T_set : Outport
  POWER_s : Outport  Port=2
  H_st : Outport  Port=3
  wires:
  Constant1/1 -> Divide1/1
  Constant2/1 -> Divide2/1
  Divide2/1 -> Divide3/1
  Constant5/1 -> Divide3/2
  Divide3/1 -> Divide1/2
  Divide1/1 -> Add1/1
  Constant6/1 -> Add2/1
  Add2/1 -> Add1/2
  dT_set/dt/1 -> Add2/2, T_set/1
  Add1/1 -> Divide4/1
  Divide4/1 -> dT_set/dt/1
  Constant7/1 -> Divide4/2
  [POWER_s] -> Divide2/2
  P/1 -> [P]
  C_l/1 -> [C_l]
  T_fi/1 -> [T_fi]
  [C_l] -> Divide5/2
  [P] -> Divide5/1
  [T_fi] -> Divide6/2
  Constant3/1 -> Divide6/1
  [H_st] -> Add3/1
  Divide6/1 -> Add3/2
  Divide5/1 -> Divide7/1
  Add3/1 -> Divide7/2
  Divide7/1 -> POWER_s/1, [POWER_s]
  Constant8/1 -> Divide8/1
  [P] -> Divide8/2
  Constant4/1 -> Add4/1
  Divide8/1 -> Add4/2
  Add4/1 -> H_st/1, [H_st]

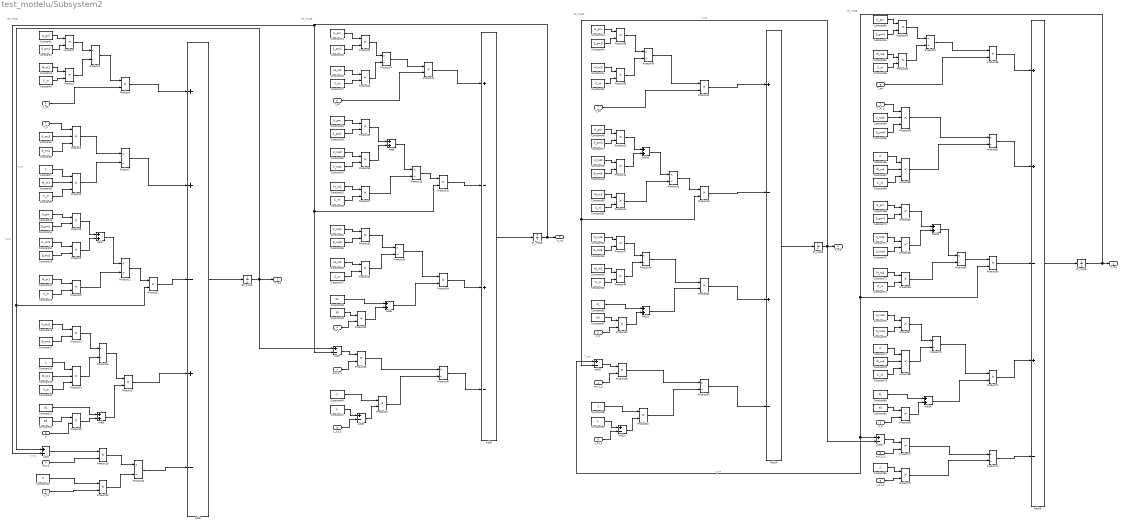
== system test_modelu/Subsystem2 ==
  note: dT_m4/dt
  note: dT_m3/dt
  note: T_m4
  note: dT_m2/dt
  note: dT_m1/dt
  note: T_m2
  T_p1 : Inport
  T_d : Inport  Port=2
  P : Inport  Port=3
  AUX1 : Inport  Port=4
  L_s1 : Inport  Port=5
  T_p2 : Inport  Port=6
  T_p3 : Inport  Port=7
  T_p4 : Inport  Port=8
  AUX1_1 : InportShadow  Port=4
  AUX1_2 : InportShadow  Port=4
  AUX1_3 : InportShadow  Port=4
  Add{1,3,5..6,10..11,15..16} (8 alike) : Sum
  Add{4,7..8,12..13,17} (6 alike) : Sum  Inputs=+-
  Add14 : Sum  Inputs=+-+-
  Add18 : Sum  Inputs=++-+-
  Add2 : Sum  Inputs=++-+-
  Add9 : Sum  Inputs=+-+-
  Constant{1,10,24,28,42,46,60,69} (8 alike) : Constant  Value=U_pm
  Constant11 : Constant  Value=S_pm1
  Constant{5,12,16,64,71,75} (6 alike) : Constant  Value=U_ms1
  Constant13 : Constant  Value=S_ms1
  Constant{3,8,14,19} (4 alike) : Constant  Value=M_m1
  Constant{4,9,15,20,27,33,37,45,51,55,63,68,74,79} (14 alike) : Constant  Value=C_m
  Constant17 : Constant  Value=S_ms1
  Constant{7,18,23,40,58,66,77,82} (8 alike) : Constant  Value=2
  Constant2 : Constant  Value=S_pm1
  Constant{21,38,56,80} (4 alike) : Constant  Value=X1
  Constant{22,39,57,81} (4 alike) : Constant  Value=K5
  Constant25 : Constant  Value=S_pm2
  Constant26 : Constant  Value=M_m2
  Constant29 : Constant  Value=S_pm2
  Constant{30,34,48,52} (4 alike) : Constant  Value=U_ms2
  Constant31 : Constant  Value=S_ms2
  Constant32 : Constant  Value=M_m2
  Constant35 : Constant  Value=S_ms2
  Constant36 : Constant  Value=M_m2
  Constant41 : Constant  Value=L
  Constant43 : Constant  Value=S_pm3
  Constant44 : Constant  Value=M_m3
  Constant47 : Constant  Value=S_pm3
  Constant49 : Constant  Value=S_ms3
  Constant50 : Constant  Value=M_m3
  Constant53 : Constant  Value=S_ms3
  Constant54 : Constant  Value=M_m3
  Constant59 : Constant  Value=L
  Constant6 : Constant  Value=S_ms1
  Constant61 : Constant  Value=S_pm4
  Constant{62,67,73,78} (4 alike) : Constant  Value=M_m4
  Constant65 : Constant  Value=S_ms4
  Constant70 : Constant  Value=S_pm4
  Constant72 : Constant  Value=S_ms4
  Constant76 : Constant  Value=S_ms4
  L_s1_1 : InportShadow  Port=5
  L_s1_2 : InportShadow  Port=5
  L_s1_3 : InportShadow  Port=5
  P_1 : InportShadow  Port=3
  P_2 : InportShadow  Port=3
  P_3 : InportShadow  Port=3
  Product{1..2,4,8..10,12..13,15,17..19,21..23,25..27,29..32,34..35,37..39,41..44,46..48,50..53,55..56,58,62..64,66..67,69,71..73} (50 alike) : Product
  Product{3,7,11,16,20,24,28,33,36,40,45,49,54,57,61,65,70,74} (18 alike) : Product  Inputs=*/
  Product{5..6,14,59..60,68} (6 alike) : Product  Inputs=3
  T_d_1 : InportShadow  Port=2
  dT_m1/dt : Integrator  InitialCondition=553.49
  dT_m2/dt : Integrator  InitialCondition=536.129
  dT_m3/dt : Integrator  InitialCondition=529.38
  dT_m4/dt : Integrator  InitialCondition=527.38
  T_m4 : Outport
  T_m1 : Outport  Port=2
  T_m2 : Outport  Port=3
  T_m3 : Outport  Port=4
  wires:
  Constant1/1 -> Product1/1
  Constant2/1 -> Product1/2
  Constant3/1 -> Product2/1
  Constant4/1 -> Product2/2
  Product1/1 -> Product3/1
  Product2/1 -> Product3/2
  T_p1/1 -> Product4/2
  Product3/1 -> Product4/1
  T_d/1 -> Product5/1
  Constant5/1 -> Product5/2
  Constant6/1 -> Product5/3
  Constant8/1 -> Product6/2
  Constant7/1 -> Product6/1
  Constant9/1 -> Product6/3
  Product5/1 -> Product7/1
  Product6/1 -> Product7/2
  Constant10/1 -> Product8/1
  Constant11/1 -> Product8/2
  Constant12/1 -> Product9/1
  Constant13/1 -> Product9/2
  Product8/1 -> Add1/1
  Product9/1 -> Add1/2
  Constant14/1 -> Product10/1
  Constant15/1 -> Product10/2
  Add1/1 -> Product11/1
  Product10/1 -> Product11/2
  Product11/1 -> Product12/1
  dT_m1/dt/1 -> Add7/1, T_m1/1, Add4/1, Product12/2  "T_m1"
  Constant16/1 -> Product13/1
  Constant17/1 -> Product13/2
  Constant19/1 -> Product14/2
  Constant18/1 -> Product14/1
  Constant20/1 -> Product14/3
  Constant21/1 -> Add3/1
  Constant22/1 -> Product15/1
  P/1 -> Product15/2
  Product13/1 -> Product16/1
  Product14/1 -> Product16/2
  Product16/1 -> Product17/1
  Add3/1 -> Product17/2
  Product4/1 -> Add2/1
  Product7/1 -> Add2/2
  Product12/1 -> Add2/3
  Product17/1 -> Add2/4
  Add4/1 -> Product18/1
  AUX1/1 -> Product18/2
  Constant23/1 -> Product19/1
  L_s1/1 -> Product19/2
  Add2/1 -> dT_m1/dt/1
  Product18/1 -> Product20/1
  Product19/1 -> Product20/2
  Product20/1 -> Add2/5
  Constant24/1 -> Product21/1
  Constant25/1 -> Product21/2
  Constant26/1 -> Product22/1
  Constant27/1 -> Product22/2
  T_p2/1 -> Product23/2
  Product21/1 -> Product24/1
  Product22/1 -> Product24/2
  Product24/1 -> Product23/1
  Constant30/1 -> Product26/1
  Constant31/1 -> Product26/2
  Constant28/1 -> Product25/1
  Constant29/1 -> Product25/2
  Constant32/1 -> Product27/1
  Constant33/1 -> Product27/2
  Product25/1 -> Add5/1
  Product26/1 -> Add5/2
  Add5/1 -> Product28/1
  Product27/1 -> Product28/2
  Product28/1 -> Product29/1
  dT_m2/dt/1 -> T_m2/1, Add4/2, Add7/2, Product29/2  "T_m2"
  Constant34/1 -> Product30/1
  Constant35/1 -> Product30/2
  Constant36/1 -> Product31/1
  Constant37/1 -> Product31/2
  Constant39/1 -> Product32/1
  P_1/1 -> Product32/2
  Constant38/1 -> Add6/1
  Product32/1 -> Add6/2
  Product15/1 -> Add3/2
  Product30/1 -> Product33/1
  Product31/1 -> Product33/2
  Product33/1 -> Product34/1
  Add6/1 -> Product34/2
  Add7/1 -> Product35/1
  AUX1_1/1 -> Product35/2
  Product35/1 -> Product36/1
  Constant41/1 -> Add8/1
  L_s1_1/1 -> Add8/2
  Constant40/1 -> Product37/1
  Add8/1 -> Product37/2
  Product37/1 -> Product36/2
  Product23/1 -> Add9/1
  Product29/1 -> Add9/2
  Product34/1 -> Add9/3
  Product36/1 -> Add9/4
  Add9/1 -> dT_m2/dt/1
  Constant42/1 -> Product38/1
  Constant43/1 -> Product38/2
  Constant44/1 -> Product39/1
  Constant45/1 -> Product39/2
  Product38/1 -> Product40/1
  Product39/1 -> Product40/2
  Product40/1 -> Product41/1
  T_p3/1 -> Product41/2
  Constant46/1 -> Product42/1
  Constant47/1 -> Product42/2
  Constant48/1 -> Product43/1
  Constant49/1 -> Product43/2
  Product42/1 -> Add10/1
  Product43/1 -> Add10/2
  Constant50/1 -> Product44/1
  Constant51/1 -> Product44/2
  Add10/1 -> Product45/1
  Product44/1 -> Product45/2
  Product45/1 -> Product46/1
  dT_m3/dt/1 -> Add17/2, Add12/2, Product46/2, T_m3/1  "T_m3"
  Constant52/1 -> Product47/1
  Constant53/1 -> Product47/2
  Constant54/1 -> Product48/1
  Constant55/1 -> Product48/2
  Product47/1 -> Product49/1
  Product48/1 -> Product49/2
  Constant57/1 -> Product50/1
  P_2/1 -> Product50/2
  Constant56/1 -> Add11/1
  Product50/1 -> Add11/2
  Product49/1 -> Product51/1
  Add11/1 -> Product51/2
  Constant59/1 -> Add13/1
  L_s1_2/1 -> Add13/2
  Constant58/1 -> Product52/1
  Add13/1 -> Product52/2
  Add12/1 -> Product53/1
  AUX1_2/1 -> Product53/2
  Product53/1 -> Product54/1
  Product52/1 -> Product54/2
  Product41/1 -> Add14/1
  Product46/1 -> Add14/2
  Product51/1 -> Add14/3
  Product54/1 -> Add14/4
  Add14/1 -> dT_m3/dt/1
  Constant60/1 -> Product55/1
  Constant61/1 -> Product55/2
  Constant62/1 -> Product56/1
  Constant63/1 -> Product56/2
  Product55/1 -> Product57/1
  Product56/1 -> Product57/2
  T_p4/1 -> Product58/2
  Product57/1 -> Product58/1
  T_d_1/1 -> Product59/1
  Constant64/1 -> Product59/2
  Constant65/1 -> Product59/3
  Constant66/1 -> Product60/1
  Constant67/1 -> Product60/2
  Constant68/1 -> Product60/3
  Product59/1 -> Product61/1
  Product60/1 -> Product61/2
  Constant69/1 -> Product62/1
  Constant70/1 -> Product62/2
  Constant71/1 -> Product63/1
  Constant72/1 -> Product63/2
  Constant73/1 -> Product64/1
  Constant74/1 -> Product64/2
  Product62/1 -> Add15/1
  Product63/1 -> Add15/2
  Add15/1 -> Product65/1
  Product64/1 -> Product65/2
  dT_m4/dt/1 -> T_m4/1, Product66/2, Add17/1, Add12/1  "T_m4"
  Product65/1 -> Product66/1
  Constant75/1 -> Product67/1
  Constant76/1 -> Product67/2
  Constant77/1 -> Product68/1
  Constant78/1 -> Product68/2
  Constant79/1 -> Product68/3
  Constant81/1 -> Product69/1
  P_3/1 -> Product69/2
  Constant80/1 -> Add16/1
  Product69/1 -> Add16/2
  Product67/1 -> Product70/1
  Product68/1 -> Product70/2
  Product70/1 -> Product71/1
  Add16/1 -> Product71/2
  Add17/1 -> Product72/1
  AUX1_3/1 -> Product72/2
  Constant82/1 -> Product73/1
  L_s1_3/1 -> Product73/2
  Product72/1 -> Product74/1
  Product73/1 -> Product74/2
  Product58/1 -> Add18/1
  Product61/1 -> Add18/2
  Product66/1 -> Add18/3
  Product71/1 -> Add18/4
  Product74/1 -> Add18/5
  Add18/1 -> dT_m4/dt/1
